simulink model "PreLab"  (R2017b)
settings: Solver=VariableStepAuto  StartTime=0.0  StopTime=10.0  RelTol=1e-3
settings Model: Creator=Ray  LastModifiedBy=Ray

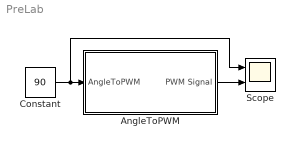
== system PreLab ==
  AngleToPWM : Subsystem
  Constant : Constant  Value=90  OutDataTypeStr=uint8  SampleTime=1
  Scope : Scope  NumInputPorts=2
  wires:
  Constant/1 -> Scope/1, AngleToPWM/1(AngleToPWM)
  AngleToPWM/1("PWM Signal ") -> Scope/2

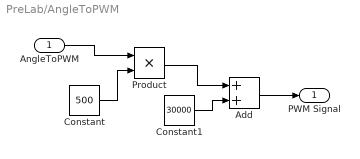
== system PreLab/AngleToPWM ==
  AngleToPWM : Inport  OutDataTypeStr=uint8  SampleTime=1
  Add : Sum  SaturateOnIntegerOverflow=on
  Constant : Constant  Value=500  SampleTime=1
  Constant1 : Constant  Value=30000  SampleTime=1
  Product : Product  SaturateOnIntegerOverflow=on
  "PWM Signal " : Outport
  wires:
  AngleToPWM/1 -> Product/1
  Constant1/1 -> Add/2
  Constant/1 -> Product/2
  Add/1 -> "PWM Signal "/1
  Product/1 -> Add/1
